simulink model "pi_controller"  (R2024a)
settings: Solver=VariableStepAuto  StartTime=0.0  StopTime=1  RelTol=1e-3
undefined symbols (not defined in the file): D, detect_delay, gear, J, K_b, K_t, Kp, L, R, taui, Ts, Wrad
settings Model: Creator=Emil  LastModifiedBy=Emil

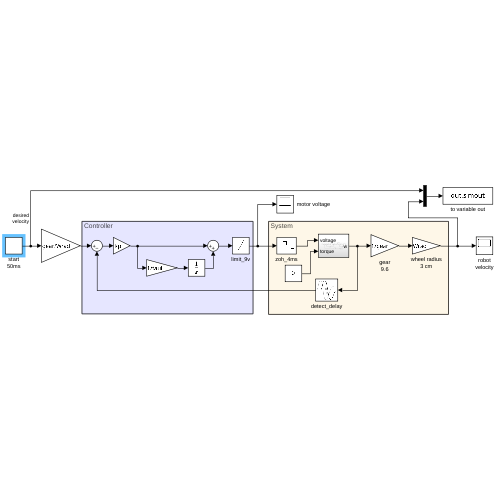
[thumbnail: Simulink's stored preview of the top-level diagram]
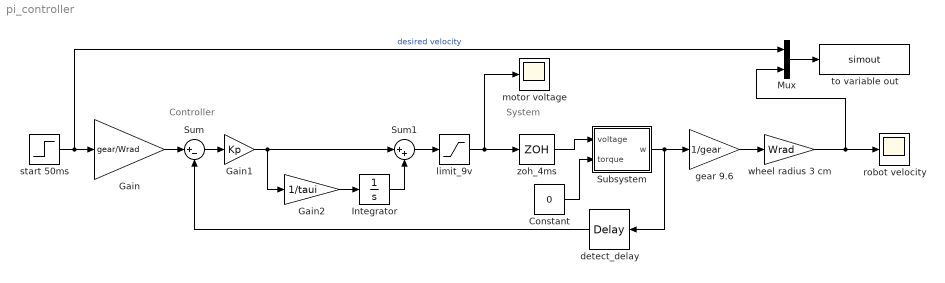
== system pi_controller ==
  note: System
  note: Controller
  Constant : Constant  Value=0
  Gain : Gain  Gain=gear/Wrad
  Gain1 : Gain  Gain=Kp
  Gain2 : Gain  Gain=1/taui
  Integrator : Integrator
  Mux : Mux  Inputs=2
  Subsystem : Subsystem
  Sum : Sum  Inputs=|+-
  Sum1 : Sum  Inputs=|++
  detect_delay : TransportDelay  DelayTime=detect_delay
  gear 9.6 : Gain  Gain=1/gear
  limit_9v : Saturate  UpperLimit=9  LowerLimit=-9
  motor voltage : Scope
  robot velocity : Scope
  start 50ms : Step  Time=0.05  SampleTime=0
  to variable out : ToWorkspace  VariableName=simout  SaveFormat=Timeseries  SampleTime=-1
  wheel radius 3 cm : Gain  Gain=Wrad
  zoh_4ms : ZeroOrderHold  SampleTime=Ts
  wires:
  start 50ms/1 -> Gain/1, Mux/1  "desired velocity"
  Gain/1 -> Sum/1
  Sum/1 -> Gain1/1
  limit_9v/1 -> zoh_4ms/1, motor voltage/1
  Subsystem/1(w) -> gear 9.6/1, detect_delay/1
  detect_delay/1 -> Sum/2
  gear 9.6/1 -> wheel radius 3 cm/1
  wheel radius 3 cm/1 -> Mux/2, robot velocity/1
  Mux/1 -> to variable out/1
  Gain2/1 -> Integrator/1
  Sum1/1 -> limit_9v/1
  Gain1/1 -> Gain2/1, Sum1/1
  Integrator/1 -> Sum1/2
  zoh_4ms/1 -> Subsystem/1(voltage)
  Constant/1 -> Subsystem/2(torque)

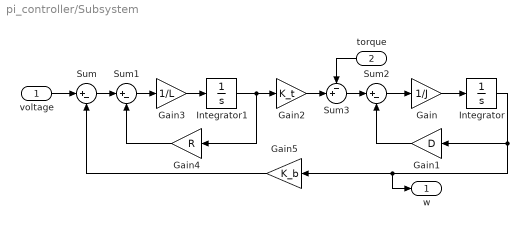
== system pi_controller/Subsystem ==
  voltage : Inport
  torque : Inport  Port=2
  Gain : Gain  Gain=1/J
  Gain1 : Gain  Gain=D
  Gain2 : Gain  Gain=K_t
  Gain3 : Gain  Gain=1/L
  Gain4 : Gain  Gain=R
  Gain5 : Gain  Gain=K_b
  Integrator : Integrator
  Integrator1 : Integrator
  Sum : Sum  Inputs=|+-
  Sum1 : Sum  Inputs=|+-
  Sum2 : Sum  Inputs=|+-
  Sum3 : Sum  Inputs=-+|
  w : Outport
  wires:
  Gain2/1 -> Sum3/2
  Gain3/1 -> Integrator1/1
  Sum/1 -> Sum1/1
  Integrator1/1 -> Gain4/1, Gain2/1
  Gain/1 -> Integrator/1
  Integrator/1 -> w/1, Gain5/1, Gain1/1
  torque/1 -> Sum3/1
  Gain1/1 -> Sum2/2
  Sum2/1 -> Gain/1
  Gain5/1 -> Sum/2
  voltage/1 -> Sum/1
  Sum1/1 -> Gain3/1
  Sum3/1 -> Sum2/1
  Gain4/1 -> Sum1/2
